simulink library "TM_MASTER"  (Simulink 8.6)
settings: Solver=ode45  StartTime=0.0  StopTime=10.0  RelTol=1e-3
libraries: cdsFilt x75, VIS_LIB x63, cdsEpicsOut x60, cdsTP x48, cdsMuxMatrix x17, cdsFiltCtrl x15, lockin x10, QPD x10, cdsRms x6, FOUROSEM_COILOUTF_MASTER x5, cdsFunctionCall x5, CRYP_TM_MASTER x3
(part 3 of 9)

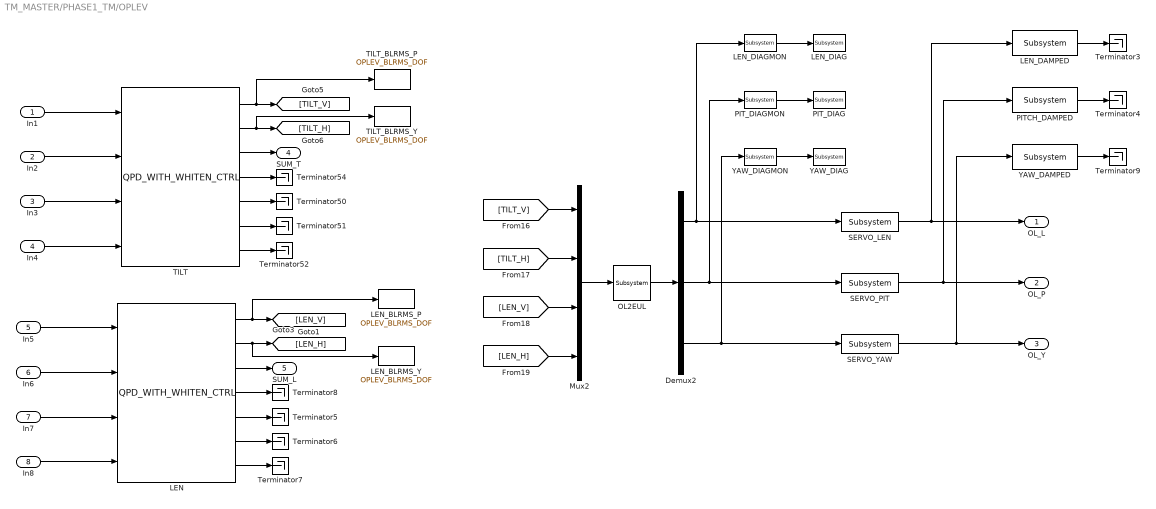
== system TM_MASTER/PHASE1_TM/OPLEV ==
  In1 : Inport
  In2 : Inport  Port=2
  In3 : Inport  Port=3
  In4 : Inport  Port=4
  In5 : Inport  Port=5
  In6 : Inport  Port=6
  In7 : Inport  Port=7
  In8 : Inport  Port=8
  Demux2 : Demux  Outputs=3
  LEN : QPD/QPD_WITH_WHITEN_CTRL
  LEN_BLRMS_P : VIS_LIB/OPLEV_BLRMS_DOF
  LEN_BLRMS_Y : VIS_LIB/OPLEV_BLRMS_DOF
  LEN_DAMPED : cdsEpicsOut/Subsystem  Tag=cdsEpicsOutput  Description=|
      | Purpose:                                          
      | Output a FE signal to an EPICS channel.           
      |                                                   
      | Operation:                                        
      | Takes input value and passes it to EPICS record.  
      |                                                   
      | Usage:                                            
      | Name the part with the desired EPICS rrecord name.
      settings: AttributesFormatString=%<Tag>
  LEN_DIAG : cdsTP/Subsystem  Tag=Test Point
      settings: AttributesFormatString=%<Tag>
  LEN_DIAGMON : cdsEpicsOut/Subsystem  Tag=cdsEpicsOutput  Description=|
      | Purpose:                                          
      | Output a FE signal to an EPICS channel.           
      |                                                   
      | Operation:                                        
      | Takes input value and passes it to EPICS record.  
      |                                                   
      | Usage:                                            
      | Name the part with the desired EPICS rrecord name.
      settings: AttributesFormatString=%<Tag>
  Mux2 : Mux
  OL2EUL : cdsMuxMatrix/Subsystem  Tag=cdsMuxMatrix  Description=Any size matrix. Inputs and outputs must be connected using Mux and Demux parts.
      settings: AttributesFormatString=%<Tag>
  PITCH_DAMPED : cdsEpicsOut/Subsystem  Tag=cdsEpicsOutput  Description=|
      | Purpose:                                          
      | Output a FE signal to an EPICS channel.           
      |                                                   
      | Operation:                                        
      | Takes input value and passes it to EPICS record.  
      |                                                   
      | Usage:                                            
      | Name the part with the desired EPICS rrecord name.
      settings: AttributesFormatString=%<Tag>
  PIT_DIAG : cdsTP/Subsystem  Tag=Test Point
      settings: AttributesFormatString=%<Tag>
  PIT_DIAGMON : cdsEpicsOut/Subsystem  Tag=cdsEpicsOutput  Description=|
      | Purpose:                                          
      | Output a FE signal to an EPICS channel.           
      |                                                   
      | Operation:                                        
      | Takes input value and passes it to EPICS record.  
      |                                                   
      | Usage:                                            
      | Name the part with the desired EPICS rrecord name.
      settings: AttributesFormatString=%<Tag>
  SERVO_LEN : cdsFilt/Subsystem  Tag=cdsFilt  Description=|
      | Purpose:                                                                                                                                                                                                                                  
      | Standard CDS IIR filter module.                                                                                                                                                                                                           
      |                                                                                                                                                                                                                                           
      | Operation:                                                                                                                                                                                                                                
      | Consists of 10 second order section IIR filters, plus a ramped gain stage. In FE code, also provides pre-defined test points and excitation channel inputs. The filter coefficients are defined in the LIGO system using the 'foton' tool.
      |                                                                                                                                                                                                                                           
      | Usage:                                                                                                                                                                                                                                    
      | Name the part with the desired filter module name.
      settings: AttributesFormatString=%<Tag>
  SERVO_PIT : cdsFilt/Subsystem  Tag=cdsFilt  Description=|
      | Purpose:                                                                                                                                                                                                                                  
      | Standard CDS IIR filter module.                                                                                                                                                                                                           
      |                                                                                                                                                                                                                                           
      | Operation:                                                                                                                                                                                                                                
      | Consists of 10 second order section IIR filters, plus a ramped gain stage. In FE code, also provides pre-defined test points and excitation channel inputs. The filter coefficients are defined in the LIGO system using the 'foton' tool.
      |                                                                                                                                                                                                                                           
      | Usage:                                                                                                                                                                                                                                    
      | Name the part with the desired filter module name.
      settings: AttributesFormatString=%<Tag>
  SERVO_YAW : cdsFilt/Subsystem  Tag=cdsFilt  Description=|
      | Purpose:                                                                                                                                                                                                                                  
      | Standard CDS IIR filter module.                                                                                                                                                                                                           
      |                                                                                                                                                                                                                                           
      | Operation:                                                                                                                                                                                                                                
      | Consists of 10 second order section IIR filters, plus a ramped gain stage. In FE code, also provides pre-defined test points and excitation channel inputs. The filter coefficients are defined in the LIGO system using the 'foton' tool.
      |                                                                                                                                                                                                                                           
      | Usage:                                                                                                                                                                                                                                    
      | Name the part with the desired filter module name.
      settings: AttributesFormatString=%<Tag>
  TILT : QPD/QPD_WITH_WHITEN_CTRL
  TILT_BLRMS_P : VIS_LIB/OPLEV_BLRMS_DOF
  TILT_BLRMS_Y : VIS_LIB/OPLEV_BLRMS_DOF
  Terminator{3..9,50..52,54} (11 alike) : Terminator
  YAW_DAMPED : cdsEpicsOut/Subsystem  Tag=cdsEpicsOutput  Description=|
      | Purpose:                                          
      | Output a FE signal to an EPICS channel.           
      |                                                   
      | Operation:                                        
      | Takes input value and passes it to EPICS record.  
      |                                                   
      | Usage:                                            
      | Name the part with the desired EPICS rrecord name.
      settings: AttributesFormatString=%<Tag>
  YAW_DIAG : cdsTP/Subsystem  Tag=Test Point
      settings: AttributesFormatString=%<Tag>
  YAW_DIAGMON : cdsEpicsOut/Subsystem  Tag=cdsEpicsOutput  Description=|
      | Purpose:                                          
      | Output a FE signal to an EPICS channel.           
      |                                                   
      | Operation:                                        
      | Takes input value and passes it to EPICS record.  
      |                                                   
      | Usage:                                            
      | Name the part with the desired EPICS rrecord name.
      settings: AttributesFormatString=%<Tag>
  OL_L : Outport
  OL_P : Outport  Port=2
  OL_Y : Outport  Port=3
  SUM_T : Outport  Port=4
  SUM_L : Outport  Port=5
  wires:
  [LEN_H] -> Mux2/4
  Mux2/1 -> OL2EUL/1
  TILT/5 -> Terminator50/1
  TILT/7 -> Terminator52/1
  TILT/6 -> Terminator51/1
  TILT/4 -> Terminator54/1
  TILT/3 -> SUM_T/1
  TILT/1 -> TILT_BLRMS_P/1, [TILT_V]
  TILT/2 -> TILT_BLRMS_Y/1, [TILT_H]
  In4/1 -> TILT/4
  In3/1 -> TILT/3
  In2/1 -> TILT/2
  In1/1 -> TILT/1
  OL2EUL/1 -> Demux2/1
  In7/1 -> LEN/3
  In6/1 -> LEN/2
  In5/1 -> LEN/1
  [LEN_V] -> Mux2/3
  LEN/3 -> SUM_L/1
  LEN/1 -> LEN_BLRMS_P/1, [LEN_V]
  In8/1 -> LEN/4
  [TILT_V] -> Mux2/1
  LEN/7 -> Terminator7/1
  LEN/6 -> Terminator6/1
  LEN/5 -> Terminator5/1
  LEN/4 -> Terminator8/1
  [TILT_H] -> Mux2/2
  Demux2/1 -> LEN_DIAGMON/1, SERVO_LEN/1
  Demux2/2 -> PIT_DIAGMON/1, SERVO_PIT/1
  Demux2/3 -> YAW_DIAGMON/1, SERVO_YAW/1
  SERVO_LEN/1 -> LEN_DAMPED/1, OL_L/1
  SERVO_PIT/1 -> PITCH_DAMPED/1, OL_P/1
  SERVO_YAW/1 -> YAW_DAMPED/1, OL_Y/1
  LEN_DAMPED/1 -> Terminator3/1
  PITCH_DAMPED/1 -> Terminator4/1
  YAW_DAMPED/1 -> Terminator9/1
  LEN/2 -> [LEN_H], LEN_BLRMS_Y/1
  LEN_DIAGMON/1 -> LEN_DIAG/1
  PIT_DIAGMON/1 -> PIT_DIAG/1
  YAW_DIAGMON/1 -> YAW_DIAG/1

== system TM_MASTER/PHASE1_TM/TEST ==
  Ground : Ground
  Ground1 : Ground
  Ground2 : Ground
  L : cdsFilt/Subsystem  Tag=cdsFilt  Description=|
      | Purpose:                                                                                                                                                                                                                                  
      | Standard CDS IIR filter module.                                                                                                                                                                                                           
      |                                                                                                                                                                                                                                           
      | Operation:                                                                                                                                                                                                                                
      | Consists of 10 second order section IIR filters, plus a ramped gain stage. In FE code, also provides pre-defined test points and excitation channel inputs. The filter coefficients are defined in the LIGO system using the 'foton' tool.
      |                                                                                                                                                                                                                                           
      | Usage:                                                                                                                                                                                                                                    
      | Name the part with the desired filter module name.
      settings: AttributesFormatString=%<Tag>
  P : cdsFilt/Subsystem  Tag=cdsFilt  Description=|
      | Purpose:                                                                                                                                                                                                                                  
      | Standard CDS IIR filter module.                                                                                                                                                                                                           
      |                                                                                                                                                                                                                                           
      | Operation:                                                                                                                                                                                                                                
      | Consists of 10 second order section IIR filters, plus a ramped gain stage. In FE code, also provides pre-defined test points and excitation channel inputs. The filter coefficients are defined in the LIGO system using the 'foton' tool.
      |                                                                                                                                                                                                                                           
      | Usage:                                                                                                                                                                                                                                    
      | Name the part with the desired filter module name.
      settings: AttributesFormatString=%<Tag>
  Y : cdsFilt/Subsystem  Tag=cdsFilt  Description=|
      | Purpose:                                                                                                                                                                                                                                  
      | Standard CDS IIR filter module.                                                                                                                                                                                                           
      |                                                                                                                                                                                                                                           
      | Operation:                                                                                                                                                                                                                                
      | Consists of 10 second order section IIR filters, plus a ramped gain stage. In FE code, also provides pre-defined test points and excitation channel inputs. The filter coefficients are defined in the LIGO system using the 'foton' tool.
      |                                                                                                                                                                                                                                           
      | Usage:                                                                                                                                                                                                                                    
      | Name the part with the desired filter module name.
      settings: AttributesFormatString=%<Tag>
  LONG_Out : Outport
  PITCH_Out : Outport  Port=2
  YAW_Out : Outport  Port=3
  wires:
  P/1 -> PITCH_Out/1
  Y/1 -> YAW_Out/1
  L/1 -> LONG_Out/1
  Ground1/1 -> P/1
  Ground/1 -> L/1
  Ground2/1 -> Y/1

== system TM_MASTER/PHASE1_TM/WD ==
  OL_T_In : Inport
  OL_L_In : Inport  Port=2
  OLAC : Subsystem
  OSEM_AC_FLAG_Out : Outport
  wires:
  OL_L_In/1 -> OLAC/2(L_In)
  OL_T_In/1 -> OLAC/1(T_In)
  OLAC/1(FLAG) -> OSEM_AC_FLAG_Out/1

== system TM_MASTER/PHASE1_TM_NEW/ADD ==
  ISC_L_In : Inport
  ISC_P_In : Inport  Port=2
  ISC_Y_In : Inport  Port=3
  TEST_L_In : Inport  Port=4
  TEST_P_In : Inport  Port=5
  TEST_Y_In : Inport  Port=6
  DAMP_L_In : Inport  Port=7
  DAMP_P_In : Inport  Port=8
  DAMP_Y_In : Inport  Port=9
  Ground{1..6} (6 alike) : Ground
  L : cdsFiltCtrl/IIR FM with control  Tag=cdsFiltCtrl  Description=|
      | cdsFiltCntrl is the standard IIR filter module (exactly the same as cdsFilt) but with added control data output 'Ctrl'. Filter module digital signal output appears on the first output, which is called 'Val'. 'Ctrl' output has a bit pattern encoding the state of filter's on/off switches (FM1 through FM10). The bit values are:
      |                                                                                                                                                                                                                                                                                                                                       
      | module 	hex	dec                                                                                                                                                                                                                                                                                                                       
      | -----------------------                                                                                                                                                                                                                                                                                                               
      | FM1	0x20                    32                                                                                                                                                                                                                                                                                                        
      | FM2	0x80                     128                                                                                                                                                                                                                                                                                                      
      | FM3	0x200                   512                                                                                                                                                                                                                                                                                                       
      | FM4	0x800                   2048                                                                                                                                                                                                                                                                                                      
      | FM5	0x2000                 8192                                                                                                                                                                                                                                                                                                       
      | FM6	0x8000                 32768                                                                                                                                                                                                                                                                                                      
      | FM7	0x20000                131072                                                                                                                                                                                                                                                                                                     
      | FM8	0x80000                 524288                                                                                                                                                                                                                                                                                                    
      | FM9	0x200000               2097152                                                                                                                                                                                                                                                                                                    
      | FM10	0x800000               8388608                                                                                                                                                                                                                                                                                                   
      |                                                                                                                                                                                                                                                                                                                                       
      | This bit data can be used to drive some other switches or it can be output using a binary I/O module.
      settings: AttributesFormatString=%<Tag>
  P : cdsFiltCtrl/IIR FM with control  Tag=cdsFiltCtrl  Description=|
      | cdsFiltCntrl is the standard IIR filter module (exactly the same as cdsFilt) but with added control data output 'Ctrl'. Filter module digital signal output appears on the first output, which is called 'Val'. 'Ctrl' output has a bit pattern encoding the state of filter's on/off switches (FM1 through FM10). The bit values are:
      |                                                                                                                                                                                                                                                                                                                                       
      | module 	hex	dec                                                                                                                                                                                                                                                                                                                       
      | -----------------------                                                                                                                                                                                                                                                                                                               
      | FM1	0x20                    32                                                                                                                                                                                                                                                                                                        
      | FM2	0x80                     128                                                                                                                                                                                                                                                                                                      
      | FM3	0x200                   512                                                                                                                                                                                                                                                                                                       
      | FM4	0x800                   2048                                                                                                                                                                                                                                                                                                      
      | FM5	0x2000                 8192                                                                                                                                                                                                                                                                                                       
      | FM6	0x8000                 32768                                                                                                                                                                                                                                                                                                      
      | FM7	0x20000                131072                                                                                                                                                                                                                                                                                                     
      | FM8	0x80000                 524288                                                                                                                                                                                                                                                                                                    
      | FM9	0x200000               2097152                                                                                                                                                                                                                                                                                                    
      | FM10	0x800000               8388608                                                                                                                                                                                                                                                                                                   
      |                                                                                                                                                                                                                                                                                                                                       
      | This bit data can be used to drive some other switches or it can be output using a binary I/O module.
      settings: AttributesFormatString=%<Tag>
  Sum : Sum  Inputs=+++
  Sum3 : Sum  Inputs=+++
  Sum4 : Sum  Inputs=+++
  Terminator1 : Terminator
  Terminator2 : Terminator
  Terminator3 : Terminator
  Y : cdsFiltCtrl/IIR FM with control  Tag=cdsFiltCtrl  Description=|
      | cdsFiltCntrl is the standard IIR filter module (exactly the same as cdsFilt) but with added control data output 'Ctrl'. Filter module digital signal output appears on the first output, which is called 'Val'. 'Ctrl' output has a bit pattern encoding the state of filter's on/off switches (FM1 through FM10). The bit values are:
      |                                                                                                                                                                                                                                                                                                                                       
      | module 	hex	dec                                                                                                                                                                                                                                                                                                                       
      | -----------------------                                                                                                                                                                                                                                                                                                               
      | FM1	0x20                    32                                                                                                                                                                                                                                                                                                        
      | FM2	0x80                     128                                                                                                                                                                                                                                                                                                      
      | FM3	0x200                   512                                                                                                                                                                                                                                                                                                       
      | FM4	0x800                   2048                                                                                                                                                                                                                                                                                                      
      | FM5	0x2000                 8192                                                                                                                                                                                                                                                                                                       
      | FM6	0x8000                 32768                                                                                                                                                                                                                                                                                                      
      | FM7	0x20000                131072                                                                                                                                                                                                                                                                                                     
      | FM8	0x80000                 524288                                                                                                                                                                                                                                                                                                    
      | FM9	0x200000               2097152                                                                                                                                                                                                                                                                                                    
      | FM10	0x800000               8388608                                                                                                                                                                                                                                                                                                   
      |                                                                                                                                                                                                                                                                                                                                       
      | This bit data can be used to drive some other switches or it can be output using a binary I/O module.
      settings: AttributesFormatString=%<Tag>
  LONG_Out : Outport
  PITCH_Out : Outport  Port=2
  YAW_Out : Outport  Port=3
  wires:
  Y/2 -> Terminator3/1
  P/2 -> Terminator2/1
  L/2 -> Terminator1/1
  Y/1 -> YAW_Out/1
  Ground5/1 -> Y/2
  Ground4/1 -> Y/3
  Sum3/1 -> Y/1
  P/1 -> PITCH_Out/1
  Ground3/1 -> P/2
  Ground2/1 -> P/3
  Sum4/1 -> P/1
  L/1 -> LONG_Out/1
  Ground6/1 -> L/2
  Ground1/1 -> L/3
  Sum/1 -> L/1
  ISC_P_In/1 -> Sum4/1
  TEST_P_In/1 -> Sum4/2
  TEST_Y_In/1 -> Sum3/2
  ISC_Y_In/1 -> Sum3/1
  TEST_L_In/1 -> Sum/2
  ISC_L_In/1 -> Sum/1
  DAMP_L_In/1 -> Sum/3
  DAMP_P_In/1 -> Sum4/3
  DAMP_Y_In/1 -> Sum3/3

== system TM_MASTER/PHASE1_TM_NEW/ADDASC ==
  ISC_P_In : Inport
  ISC_Y_In : Inport  Port=2
  DITHER_P_In : Inport  Port=3
  DITHER_Y_In : Inport  Port=4
  Sum3 : Sum
  Sum4 : Sum
  PITCH_Out : Outport
  YAW_Out : Outport  Port=2
  wires:
  Sum3/1 -> YAW_Out/1
  ISC_P_In/1 -> Sum4/1
  ISC_Y_In/1 -> Sum3/1
  Sum4/1 -> PITCH_Out/1
  DITHER_P_In/1 -> Sum4/2
  DITHER_Y_In/1 -> Sum3/2
